simulink model "clik_inverse"  (R2021b)
settings: Solver=ode1  StartTime=0.0  StopTime=4  FixedStep=0.001  RelTol=1e-3
undefined symbols (not defined in the file or in its folder): DiscIntNeverNeededParam, q0
settings Model: Creator=Xp  LastModifiedBy=rajat
settings SolverCC: AlgebraicLoopSolver=TrustRegion
settings DataIOCC: LimitDataPoints=on  SaveFormat=Array  SignalLoggingSaveFormat=ModelDataLogs  ReturnWorkspaceOutputs=off
settings OptimizationCC: ExpressionDepthLimit=2147483647  InitFltsAndDblsToZero=on  LifeSpan=inf
settings DebuggingCC: SaveWithParameterizedLinksMsg=none  UnderspecifiedInitializationDetection=Classic  MergeDetectMultiDrivingBlocksExec=none  SolverPrmCheckMsg=warning  MultiTaskDSMMsg=warning  MultiTaskCondExecSysMsg=none  FcnCallInpInsideContextMsg=warning  StateNameClashWarn=warning  SFUnexpectedBacktrackingDiag=warning  SFNoUnconditionalDefaultTransitionDiag=warning  SFExecutionAtInitializationDiag=none  SFMachineParentedDataDiag=warning  ArithmeticOperatorsInVariantConditions=warning
settings HardwareCC: ProdBitPerPointer=32  ProdBitPerSizeT=32  ProdBitPerPtrDiffT=32  ProdLargestAtomicFloat=None  ProdIntDivRoundTo=Undefined  ProdEndianess=Unspecified  ProdWordSize=32  ProdHWDeviceType=32-bit Generic
settings ModelReferenceCC: PropagateSignalLabelsOutOfModel=off
settings SFSimCC: CustomCodeUndefinedFunction=UseInterfaceOnly
settings CodeAppCC: StateflowObjectComments=on
settings GRTTargetCC: TargetLangStandard=C89/C90 (ANSI)  CombineOutputUpdateFcns=off  GRTInterface=on
settings ConfigComp: CovMetricSettings=dw  CovSaveCumulativeToWorkspaceVar=on  CovSaveSingleToWorkspaceVar=on

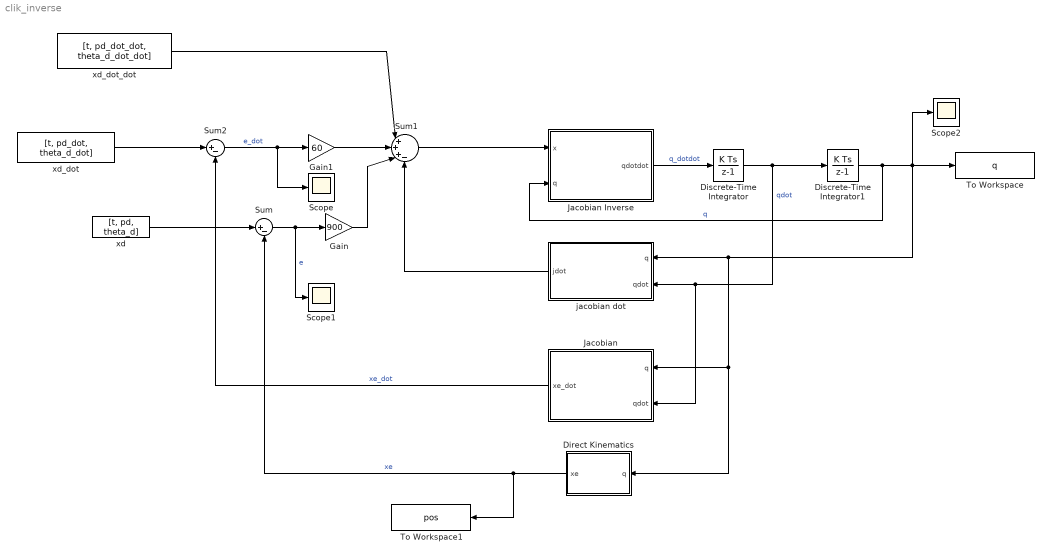
== system clik_inverse ==
  Direct Kinematics : MATLAB Function  TreatAsAtomicUnit=on
  Discrete-Time Integrator : DiscreteIntegrator  InitialCondition=[0;0;0;0]  SampleTime=0.001  ICPrevOutput=DiscIntNeverNeededParam  ICPrevScaledInput=DiscIntNeverNeededParam
  Discrete-Time Integrator1 : DiscreteIntegrator  InitialCondition=q0  SampleTime=0.001  LimitOutput=on  UpperSaturationLimit=[pi/2;pi/4;1;2*pi]  LowerSaturationLimit=[-pi/2;-pi/2;0.25;-2*pi]  ICPrevOutput=DiscIntNeverNeededParam  ICPrevScaledInput=DiscIntNeverNeededParam
  Gain : Gain  Gain=900
  Gain1 : Gain  Gain=60
  "Jacobian " : MATLAB Function  TreatAsAtomicUnit=on
  Jacobian Inverse : MATLAB Function  TreatAsAtomicUnit=on
  Scope : Scope
  Scope1 : Scope
  Scope2 : Scope
  Sum : Sum  Inputs=|+-
  Sum1 : Sum  Inputs=|+++-
  Sum2 : Sum  Inputs=|+-
  To Workspace : ToWorkspace  VariableName=q  SampleTime=0.001
  To Workspace1 : ToWorkspace  VariableName=pos  SampleTime=0.001
  jacobian dot : MATLAB Function  TreatAsAtomicUnit=on
  xd : FromWorkspace  VariableName=[t, pd, theta_d]  OutDataTypeStr=double  SampleTime=0.001
  xd_dot : FromWorkspace  VariableName=[t, pd_dot, theta_d_dot]  OutDataTypeStr=double  SampleTime=0.001
  xd_dot_dot : FromWorkspace  VariableName=[t, pd_dot_dot, theta_d_dot_dot]  OutDataTypeStr=double  SampleTime=0.001
  wires:
  Direct Kinematics/1(xe) -> To Workspace1/1, Sum/2  "xe"
  Jacobian Inverse/1(qdotdot) -> Discrete-Time Integrator/1  "q_dotdot"
  Discrete-Time Integrator/1 -> "Jacobian "/2(qdot), jacobian dot/2(qdot), Discrete-Time Integrator1/1  "qdot"
  Discrete-Time Integrator1/1 -> Jacobian Inverse/2(q), Scope2/1, jacobian dot/1(q), Direct Kinematics/1(q), "Jacobian "/1(q), To Workspace/1  "q"
  xd/1 -> Sum/1
  Gain1/1 -> Sum1/2
  xd_dot_dot/1 -> Sum1/1
  Sum1/1 -> Jacobian Inverse/1(x)
  xd_dot/1 -> Sum2/1
  Sum2/1 -> Scope/1, Gain1/1  "e_dot"
  "Jacobian "/1(xe_dot) -> Sum2/2  "xe_dot"
  Sum/1 -> Scope1/1, Gain/1  "e"
  Gain/1 -> Sum1/3
  jacobian dot/1(jdot) -> Sum1/4

== matlab function clik_inverse/Jacobian Inverse ==
  data: x input; q input; qdotdot output
function qdotdot = jacobian_inverse(x,q)
qdotdot = [0;0;0;0];
qdotdot = jacobian_inverse(x,q);
end

== matlab function clik_inverse/Direct Kinematics ==
  data: q input; xe output
function xe = direct_kin(q)
xe = [0 0 0 0];
xe = direct_kin(q);
end

== matlab function clik_inverse/Jacobian  ==
  data: q input; qdot input; xe_dot output
function xe_dot  = Jacobian(q,qdot)

[~,xe_dot]  = Jacobian(q,qdot);

end

== matlab function clik_inverse/jacobian dot ==
  data: q input; jdot output; qdot input
function jdot = jacobian_dot(q,qdot)
jdot = jacobian_dot(q,qdot);
end
